simulink model "tms_model"  (R2022a)
settings: Solver=VariableStepAuto  StartTime=0.0  StopTime=10.0  RelTol=1e-3
libraries: simulink x4
settings Model: Creator=schro  LastModifiedBy=schro

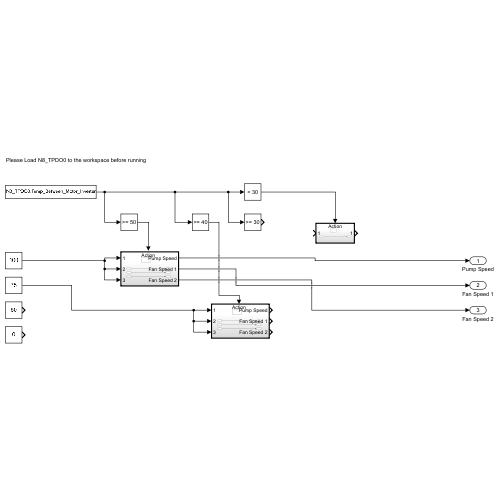
[thumbnail: Simulink's stored preview of the top-level diagram]
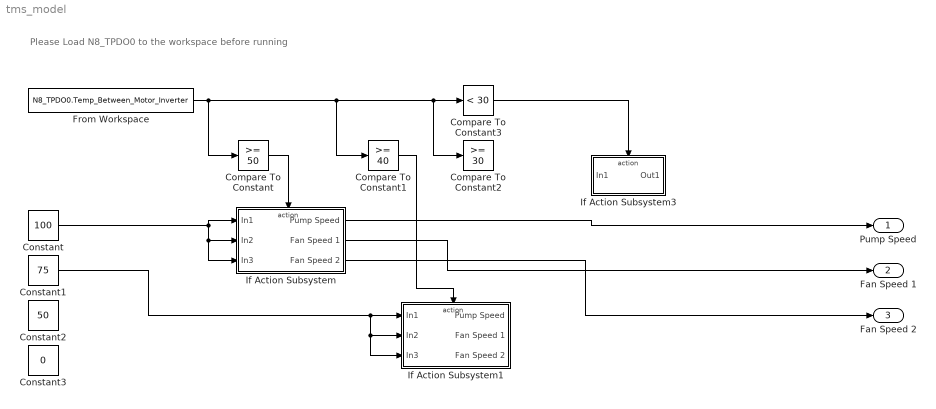
== system tms_model ==
  note: Please Load N8_TPDO0 to the workspace before running
  Compare To Constant : simulink/Logic and Bit Operations/Compare To Constant  relop=>=  const=50  OutDataTypeStr=boolean
  Compare To Constant1 : simulink/Logic and Bit Operations/Compare To Constant  relop=>=  const=40  OutDataTypeStr=boolean
  Compare To Constant2 : simulink/Logic and Bit Operations/Compare To Constant  relop=>=  const=30  OutDataTypeStr=boolean
  Compare To Constant3 : simulink/Logic and Bit Operations/Compare To Constant  relop=<  const=30  OutDataTypeStr=boolean
  Constant : Constant  Value=100
  Constant1 : Constant  Value=75
  Constant2 : Constant  Value=50
  Constant3 : Constant  Value=0
  From Workspace : FromWorkspace  VariableName=N8_TPDO0.Temp_Between_Motor_Inverter
  If Action Subsystem : Subsystem  TreatAsAtomicUnit=on
  If Action Subsystem1 : Subsystem  TreatAsAtomicUnit=on
  If Action Subsystem3 : Subsystem  TreatAsAtomicUnit=on
  Pump Speed : Outport
  Fan Speed 1 : Outport  Port=2
  Fan Speed 2 : Outport  Port=3
  wires:
  From Workspace/1 -> Compare To Constant1/1, Compare To Constant3/1, Compare To Constant2/1, Compare To Constant/1
  Compare To Constant3/1 -> If Action Subsystem3/Action
  Compare To Constant/1 -> If Action Subsystem/Action
  Constant/1 -> If Action Subsystem/3(In3), If Action Subsystem/2(In2), If Action Subsystem/1(In1)
  If Action Subsystem/1(Pump Speed) -> Pump Speed/1
  If Action Subsystem/3(Fan Speed 2) -> Fan Speed 2/1
  If Action Subsystem/2(Fan Speed 1) -> Fan Speed 1/1
  Compare To Constant1/1 -> If Action Subsystem1/Action
  Constant1/1 -> If Action Subsystem1/3(In3), If Action Subsystem1/2(In2), If Action Subsystem1/1(In1)

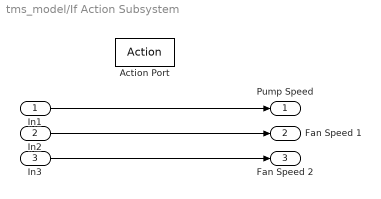
== system tms_model/If Action Subsystem ==
  In1 : Inport
  In2 : Inport  Port=2
  In3 : Inport  Port=3
  Action Port : ActionPort
  Pump Speed : Outport
  Fan Speed 1 : Outport  Port=2
  Fan Speed 2 : Outport  Port=3
  wires:
  In1/1 -> Pump Speed/1
  In2/1 -> Fan Speed 1/1
  In3/1 -> Fan Speed 2/1

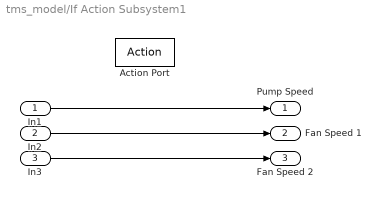
== system tms_model/If Action Subsystem1 ==
  In1 : Inport
  In2 : Inport  Port=2
  In3 : Inport  Port=3
  Action Port : ActionPort
  Pump Speed : Outport
  Fan Speed 1 : Outport  Port=2
  Fan Speed 2 : Outport  Port=3
  wires:
  In1/1 -> Pump Speed/1
  In2/1 -> Fan Speed 1/1
  In3/1 -> Fan Speed 2/1

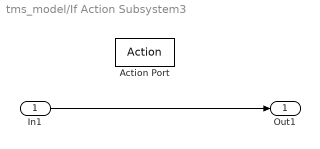
== system tms_model/If Action Subsystem3 ==
  In1 : Inport
  Action Port : ActionPort
  Out1 : Outport
  wires:
  In1/1 -> Out1/1
